simulink library "WavePlayLibBtc"  (R2022b)
settings: Solver=VariableStepAuto  StartTime=0.0  StopTime=10.0  RelTol=1e-3
values from neighbouring files (symbols this model uses):
  selectclickclack = 1    [chimes_init.m]
  TotalPeriod = 25    [chimes_init.m]
undefined symbols (not defined in the file or in its folder): Row
libraries: TuneVar x8, TOP x4, FeaturePath x1, HandyTextFile x1, RTC x1
settings Model: Creator=kl13806  LastModifiedBy=kl13806
settings SolverCC: AlgebraicLoopSolver=TrustRegion
settings DebuggingCC: UnconnectedInputMsg=warning  UnconnectedOutputMsg=warning  UnconnectedLineMsg=warning  SFMachineParentedDataDiag=warning
settings ModelReferenceCC: EnableRefExpFcnMdlSchedulingChecks=on
settings RTWCC: DLArmComputeVersion=19.05

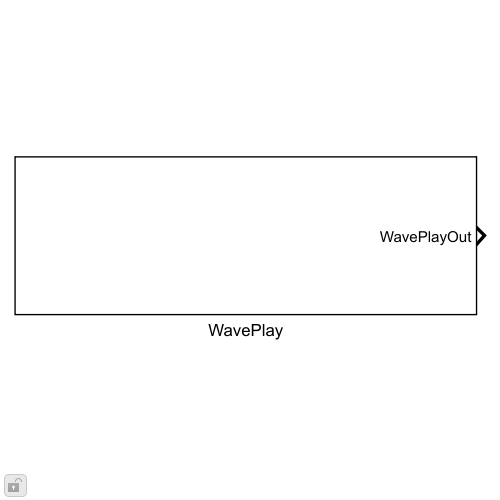
[thumbnail: Simulink's stored preview of the top-level diagram]
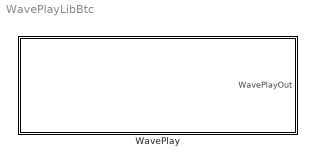
== system WavePlayLibBtc ==
  WavePlay : Subsystem  mask(Chimes WavePlay){Config=[], FeatureName=Waveplay}
      mask prompts: Config "WavePlayConfig"; FeatureName "Feature path name:"
      mask help:
      | % DESCRIPTION:
      |  Waveplay is a single-channel wave player that plays out stored waveforms.
      |   p.playControl        -  Volume and switch to start wave play
      |   p.controlState       -   Old state of playControl
      |   p.frameSize           -   Frame size
      |   p.tableLength       -   Length of the wave table
      |   p.table                   -    Wave table
      |   p.tableIndex         -    Index into wave table
      |   minVol                  -    Trigger threshold for waveplay
      mask init:
      | blkh=gcbh;
      | Config=BTConfig.Assert(blkh,Config);
      | Config.Validate();
      | BTConfig.InitSetFeatureIfPresent(blkh,'FeatureName');
      mask Callback Config: BTConfig.CallbackHideIfPresent(gcbh,{'FeatureName'});
      mask TypeOptions FeatureName: FeaturePath/FeatureName

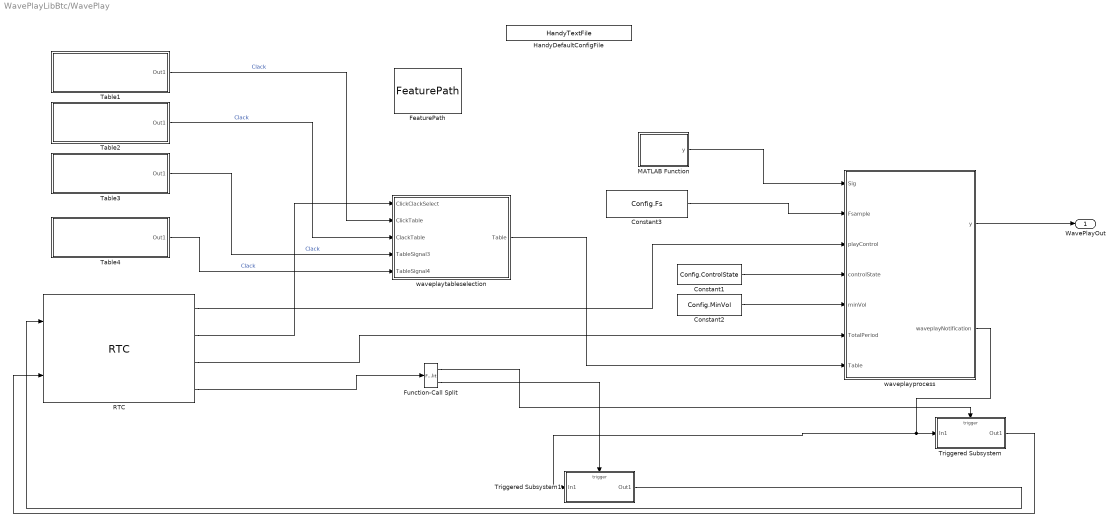
== system WavePlayLibBtc/WavePlay ==
  Constant1 : Constant  Value=Config.ControlState  OutDataTypeStr=single
  Constant2 : Constant  Value=Config.MinVol  OutDataTypeStr=single
  Constant3 : Constant  Value=Config.Fs
  FeaturePath : FeaturePath/FeaturePath  FeatureName=Waveplay  IsGroup=off  GroupNumber=-1  IsModule=off  TriggerInit=[885 274 985 341]
      settings: SourceProductName=Bose Talaria
  Function-Call Split : FunctionCallSplit  IconShape=distinctive  NumOutputPorts=2  OutputPortLayout=default
  HandyDefaultConfigFile : HandyTextFile/HandyTextFile  TemplateSource=Config  FileSuffix=Init  OpenDialogOnLoad=off  UseThisBlockName=off  AddGrandParentNamePrefix=off  TheDefaultText=|  ShowInLibBrowser=on
      | % $(FILENAME) Setup model parameters for each "Init" callback (e.g. update diagram)
      | sample_rate_in_hertz = 44100;
      | frame_size = 32;
      | sysin_channel_count = 2;
      settings: SourceProductName=Bose Talaria
  MATLAB Function : MATLAB Function  TreatAsAtomicUnit=on  mask{frameSize=Config.FrameSize}
  RTC : RTC/RTC  REQ_Priority=RTC_Mask.NormalPriority  RequestAtInit=off  EnableRequest=off  REQElemName1=WavePlayControl  REQElemType1=single  REQElemWidth1=length(Config.InitialPlayControl)  REQElemInitial1=Config.InitialPlayControl  REQElemName2=ClickClackSelect  REQElemType2=uint32  REQElemWidth2=length(selectclickclack)  REQElemInitial2=Config.InitialClickClackSelect  REQElemName3=TotalPeriod  REQElemType3=single  REQElemWidth3=length(TotalPeriod)  REQElemInitial3=Config.InitialTotalPeriodMsec  REQElemType4=uint32  REQElemWidth4=1  REQElemInitial4=[]  REQElemType5=uint32  REQElemWidth5=1  REQElemInitial5=[]  REQElemType6=uint32  REQElemWidth6=1  REQElemInitial6=[]  REQElemType7=uint32  REQElemWidth7=1  REQElemInitial7=[]  REQElemType8=uint32  REQElemWidth8=1  REQElemInitial8=[]  REQElemType9=uint32  REQElemWidth9=1  REQElemInitial9=[]  REQElemType10=uint32  REQElemWidth10=1  REQElemInitial10=[]  EnableResponse=on  EnableRSP_StatusIn=off  RSPElemType1=uint32  RSPElemWidth1=1  RSPElemType2=uint32  RSPElemWidth2=1  RSPElemType3=uint32  RSPElemWidth3=1  RSPElemType4=uint32  RSPElemWidth4=1  RSPElemType5=uint32  RSPElemWidth5=1  RSPElemType6=uint32  RSPElemWidth6=1  RSPElemType7=uint32  RSPElemWidth7=1  RSPElemType8=uint32  RSPElemWidth8=1  RSPElemType9=uint32  RSPElemWidth9=1  RSPElemType10=uint32  RSPElemWidth10=1  EnableNotification=on  EnableNTF_PrepTrig=off  NTFElemName1=WaveplayDone  NTFElemType1=uint32  NTFElemWidth1=1  NTFElemType2=uint32  NTFElemWidth2=1  NTFElemType3=uint32  NTFElemWidth3=1  NTFElemType4=uint32  NTFElemWidth4=1  NTFElemType5=uint32  NTFElemWidth5=1  NTFElemType6=uint32  NTFElemWidth6=1  NTFElemType7=uint32  NTFElemWidth7=1  NTFElemType8=uint32  NTFElemWidth8=1  NTFElemType9=uint32  NTFElemWidth9=1  NTFElemType10=uint32  NTFElemWidth10=1  MaskMessageName=RTC
      settings: SourceProductName=Bose Talaria
  Table1 : Subsystem
  Table2 : Subsystem
  Table3 : Subsystem
  Table4 : Subsystem
  Triggered Subsystem : Subsystem  TreatAsAtomicUnit=on
  Triggered Subsystem1 : Subsystem  TreatAsAtomicUnit=on
  waveplayprocess : MATLAB Function  TreatAsAtomicUnit=on
  waveplaytableselection : MATLAB Function  TreatAsAtomicUnit=on
  WavePlayOut : Outport  VectorParamsAs1DForOutWhenUnconnected=off
  wires:
  waveplayprocess/1(y) -> WavePlayOut/1
  Constant1/1 -> waveplayprocess/4(controlState)
  RTC/1 -> waveplayprocess/3(playControl)
  Constant2/1 -> waveplayprocess/5(minVol)
  Triggered Subsystem/1(Out1) -> RTC/2
  waveplayprocess/2(waveplayNotification) -> Triggered Subsystem1/1(In1), Triggered Subsystem/1(In1)
  Triggered Subsystem1/1(Out1) -> RTC/1
  RTC/4 -> Function-Call Split/1
  Function-Call Split/1 -> Triggered Subsystem/Trigger
  Function-Call Split/2 -> Triggered Subsystem1/Trigger
  Constant3/1 -> waveplayprocess/2(Fsample)
  RTC/2 -> waveplaytableselection/1(ClickClackSelect)
  Table1/1(Out1) -> waveplaytableselection/2(ClickTable)  "Clack"
  Table2/1(Out1) -> waveplaytableselection/3(ClackTable)  "Clack"
  Table3/1(Out1) -> waveplaytableselection/4(TableSignal3)  "Clack"
  Table4/1(Out1) -> waveplaytableselection/5(TableSignal4)  "Clack"
  waveplaytableselection/1(Table) -> waveplayprocess/7(Table)
  RTC/3 -> waveplayprocess/6(TotalPeriod)
  MATLAB Function/1(y) -> waveplayprocess/1(Sig)

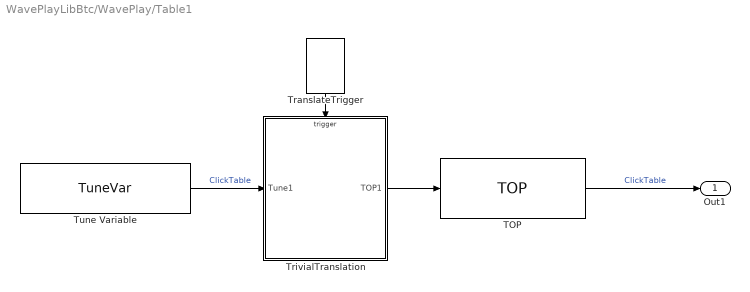
== system WavePlayLibBtc/WavePlay/Table1 ==
  TOP : TOP/TOP  TriggerInit=[440 20 585 80]  TopName=ClickTable  DataType=single  BankNumber=0  PreOverlay=false  PostOverlay=false  Role=Automatic
      settings: SourceProductName=Bose Talaria
  TranslateTrigger : TuneVar/TranslateTrigger  TriggerInit=[306 -100 344 -45]
      settings: SourceProductName=Bose Talaria
  TrivialTranslation : MATLAB Function  TreatAsAtomicUnit=on  mask(Talaria Translation){}
      mask help: This MATLAB Function Block can be automatically inserted by several automation routines. Once placed, the block is ready to accept translation logic from the model designer.
  Tune Variable : TuneVar/TuneVar  TuneName=ClickTable  SpecifyMaxSize=on  VariableDim=1 (Row)  MaxSize=[Config.MaxTableSamples 1]  TunabilityNumber=1  MinValue=[]  MaxValue=[]  TriggerInit=[20 25 190 75]  MaskValue=Config.DefaultTable1
      settings: SourceProductName=Bose Talaria
  Out1 : Outport  VectorParamsAs1DForOutWhenUnconnected=off
  wires:
  TOP/1 -> Out1/1  "ClickTable"
  Tune Variable/1 -> TrivialTranslation/1(Tune1)  "ClickTable"
  TrivialTranslation/1(TOP1) -> TOP/1
  TranslateTrigger/1 -> TrivialTranslation/Trigger

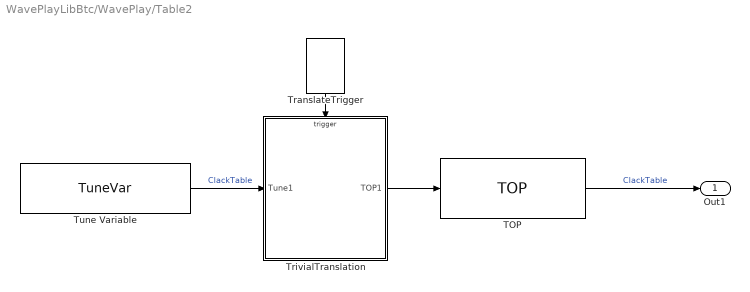
== system WavePlayLibBtc/WavePlay/Table2 ==
  TOP : TOP/TOP  TriggerInit=[440 20 585 80]  TopName=ClackTable  DataType=single  BankNumber=0  PreOverlay=false  PostOverlay=false  Role=Automatic
      settings: SourceProductName=Bose Talaria
  TranslateTrigger : TuneVar/TranslateTrigger  TriggerInit=[306 -100 344 -45]
      settings: SourceProductName=Bose Talaria
  TrivialTranslation : MATLAB Function  TreatAsAtomicUnit=on  mask(Talaria Translation){}
      mask help: This MATLAB Function Block can be automatically inserted by several automation routines. Once placed, the block is ready to accept translation logic from the model designer.
  Tune Variable : TuneVar/TuneVar  TuneName=ClackTable  SpecifyMaxSize=on  VariableDim=1 (Row)  MaxSize=[Config.MaxTableSamples 1]  TunabilityNumber=1  MinValue=[]  MaxValue=[]  TriggerInit=[20 25 190 75]  MaskValue=Config.DefaultTable2
      settings: SourceProductName=Bose Talaria
  Out1 : Outport  VectorParamsAs1DForOutWhenUnconnected=off
  wires:
  TOP/1 -> Out1/1  "ClackTable"
  Tune Variable/1 -> TrivialTranslation/1(Tune1)  "ClackTable"
  TrivialTranslation/1(TOP1) -> TOP/1
  TranslateTrigger/1 -> TrivialTranslation/Trigger

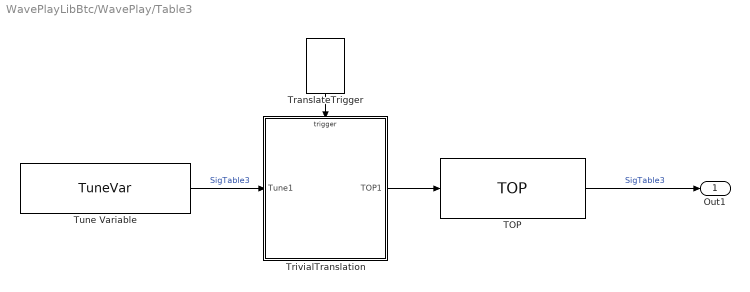
== system WavePlayLibBtc/WavePlay/Table3 ==
  TOP : TOP/TOP  TriggerInit=[440 20 585 80]  TopName=SigTable3  DataType=single  BankNumber=0  PreOverlay=false  PostOverlay=false  Role=Automatic
      settings: SourceProductName=Bose Talaria
  TranslateTrigger : TuneVar/TranslateTrigger  TriggerInit=[306 -100 344 -45]
      settings: SourceProductName=Bose Talaria
  TrivialTranslation : MATLAB Function  TreatAsAtomicUnit=on  mask(Talaria Translation){}
      mask help: This MATLAB Function Block can be automatically inserted by several automation routines. Once placed, the block is ready to accept translation logic from the model designer.
  Tune Variable : TuneVar/TuneVar  TuneName=SigTable3  SpecifyMaxSize=on  VariableDim=1 (Row)  MaxSize=[Config.MaxTableSamples 1]  TunabilityNumber=1  MinValue=[]  MaxValue=[]  TriggerInit=[20 25 190 75]  MaskValue=Config.DefaultTable3
      settings: SourceProductName=Bose Talaria
  Out1 : Outport  VectorParamsAs1DForOutWhenUnconnected=off
  wires:
  TOP/1 -> Out1/1  "SigTable3"
  Tune Variable/1 -> TrivialTranslation/1(Tune1)  "SigTable3"
  TrivialTranslation/1(TOP1) -> TOP/1
  TranslateTrigger/1 -> TrivialTranslation/Trigger

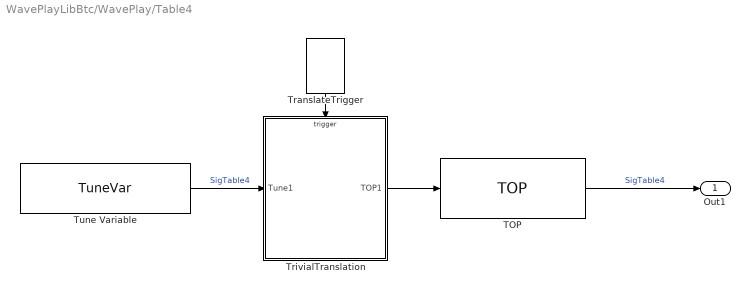
== system WavePlayLibBtc/WavePlay/Table4 ==
  TOP : TOP/TOP  TriggerInit=[440 20 585 80]  TopName=SigTable4  DataType=single  BankNumber=0  PreOverlay=false  PostOverlay=false  Role=Automatic
      settings: SourceProductName=Bose Talaria
  TranslateTrigger : TuneVar/TranslateTrigger  TriggerInit=[306 -100 344 -45]
      settings: SourceProductName=Bose Talaria
  TrivialTranslation : MATLAB Function  TreatAsAtomicUnit=on  mask(Talaria Translation){}
      mask help: This MATLAB Function Block can be automatically inserted by several automation routines. Once placed, the block is ready to accept translation logic from the model designer.
  Tune Variable : TuneVar/TuneVar  TuneName=SigTable4  SpecifyMaxSize=on  VariableDim=1 (Row)  MaxSize=[Config.MaxTableSamples 1]  TunabilityNumber=1  MinValue=[]  MaxValue=[]  TriggerInit=[20 25 190 75]  MaskValue=Config.DefaultTable4
      settings: SourceProductName=Bose Talaria
  Out1 : Outport  VectorParamsAs1DForOutWhenUnconnected=off
  wires:
  TOP/1 -> Out1/1  "SigTable4"
  Tune Variable/1 -> TrivialTranslation/1(Tune1)  "SigTable4"
  TrivialTranslation/1(TOP1) -> TOP/1
  TranslateTrigger/1 -> TrivialTranslation/Trigger

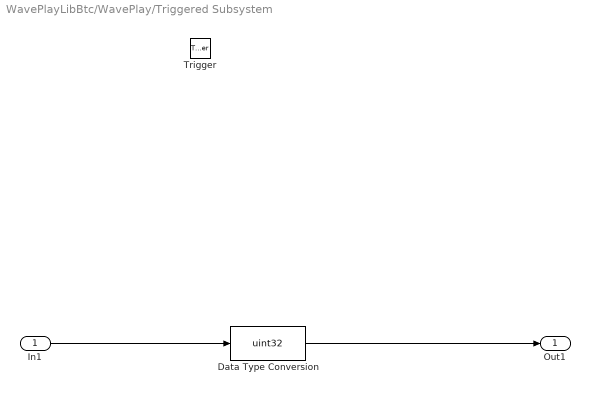
== system WavePlayLibBtc/WavePlay/Triggered Subsystem ==
  In1 : Inport
  Trigger : TriggerPort  TriggerType=function-call  VariantControl=Variant
  Data Type Conversion : DataTypeConversion  OutDataTypeStr=uint32  SaturateOnIntegerOverflow=off  RndMeth=Floor
  Out1 : Outport
  wires:
  In1/1 -> Data Type Conversion/1
  Data Type Conversion/1 -> Out1/1

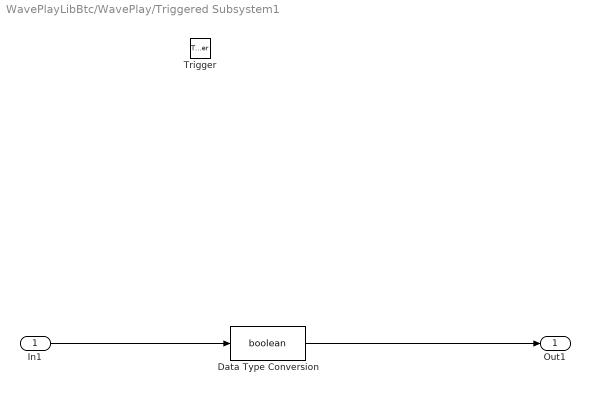
== system WavePlayLibBtc/WavePlay/Triggered Subsystem1 ==
  In1 : Inport
  Trigger : TriggerPort  TriggerType=function-call  VariantControl=Variant
  Data Type Conversion : DataTypeConversion  OutDataTypeStr=boolean  SaturateOnIntegerOverflow=off  RndMeth=Floor
  Out1 : Outport
  wires:
  Data Type Conversion/1 -> Out1/1
  In1/1 -> Data Type Conversion/1

== matlab function WavePlayLibBtc/WavePlay/waveplaytableselection ==
  data: ClickClackSelect input; Table output; ClickTable input; ClackTable input; TableSignal3 input; TableSignal4 input
function Table  = fcn(ClickClackSelect,ClickTable,ClackTable,TableSignal3,TableSignal4)
    
   MaxTableLen=single(1120.0);    
   Table = single(zeros(MaxTableLen,1));
%% Note : Maximum Table length number has been chosen based on use case of click and clack
%         signals, typically click signal is of 1079 values, and clack signal is of
%         1095 values, we round off to the nearest number in multiple of frame size.
    switch(ClickClackSelect)
        case 1 %% Click signal table selection
            Table = ClickTable;
        case 2 %% Clack signal table selection
            Table = ClackTable;
        case 3 %% Table3 signal table selection
            Table = TableSignal3;
        case 4 %% Table4 signal table selection
            Table = TableSignal4;          
    end

== matlab function WavePlayLibBtc/WavePlay/waveplayprocess ==
  data: Sig input; Fsample input; y output size=[32 1]; playControl input; controlState input; minVol input; TotalPeriod input; waveplayNotification output; Table input
function [y,waveplayNotification] = fcn(Sig,Fsample,playControl,controlState,minVol,TotalPeriod,Table)

    FrmSize= single(size(Sig,1));
    Fsamp= Fsample(1,1);
    
    waveplayNotification =single(0.0);
    persistent OutStore ;
    persistent waveplayDone;
    persistent ctlState;
    persistent tableIndex;
    persistent SilencePeriodCounter;
    Numchannels = size(Table,2);
    tableLength = size(Table,1);
    TablePeriod = (tableLength/Fsamp)*1000;
    quantum_ms  = 1000 * FrmSize / Fsamp;
    SilencePeriod= TotalPeriod - TablePeriod;
    
    if(isempty(OutStore))
        SilencePeriodCounter = ceil(SilencePeriod/quantum_ms);
    end

    if(isempty(OutStore))
         OutStore = single(zeros(FrmSize,Numchannels));        
    end
    if(isempty(ctlState))
        ctlState = controlState;% single(0.0);
    end
    if(isempty(tableIndex))
        tableIndex = single(0.0);
    end
    if(isempty(waveplayDone))
        waveplayDone =single(0.0);
    end
    
    if (playControl < minVol)    % playControl == 0
        OutStore(:,1:Numchannels) = zeros(FrmSize, 1);   
    else                           % playControl ~= 0
    % start wave play at the rising edge of playControl signal
    % assuming p has been properly initialized before rising edge occurs
        if((playControl - ctlState) > minVol)      % trigger detected
            % playControl also acts as playing volume     
            OutStore(:,1:Numchannels) = playControl .* Table(1:FrmSize);
            tableIndex = FrmSize;  % update tabelIndex after outputing the 1st frame
        else       %  playControl = controlState (both >= minVol)
            i = tableIndex;
            %if(i >= tableLength)
            if((tableLength-tableIndex)<FrmSize)
                %We do reset here, compared to BDSP implementation
                tableIndex = single(0.0);
                waveplayDone=single(1.0);
                i=single(0.0);
            end
            if (i < tableLength)   % continuation frame
                OutStore(:,1:Numchannels) = playControl .* Table(i+1:i+FrmSize);
                tableIndex = i + FrmSize;   % don't wrap around, o/w, next condition won't be met
            else        % i >= p.tableLength, wave table done
                OutStore(:,1:Numchannels) = zeros(FrmSize, 1);   
                % don't update tableIndex to keep the condition "i >= tableLength" valid
                % TableIndex will be reset when next trigger arrives
            end  
        end
   end
    ctlState = playControl;   % save previous state
    if(waveplayDone)
        %This is a wrap around case when table is finished,if we have
        %silent period>0 then only we send zeros to microcontroller
        %otherwise we need to wrap around to table values after we complete
        %reading table 
        if(SilencePeriodCounter>0)% To avoid boundary condition
            SilencePeriodCounter=SilencePeriodCounter-1;
            OutStore(:,1:Numchannels) = zeros(FrmSize, 1);
            tableIndex = single(0.0);
        end
      if(~SilencePeriodCounter)
        waveplayDone=single(0.0);  
        %Now that we are done with check of click/clack table finished,
        %And also the silence period is completed,notify to micro.
        waveplayNotification =single(1.0);
        SilencePeriodCounter = ceil(SilencePeriod/quantum_ms);        
      end
    end %% waveplayDone
 y = OutStore;

== matlab function WavePlayLibBtc/WavePlay/MATLAB Function ==
  data: y output size=[frameSize 1]; frameSize parameter
function y = fcn(frameSize)
% zero padding 
y = zeros(frameSize,1);

== matlab function WavePlayLibBtc/WavePlay/Table2/TrivialTranslation ==
  data: TOP1 output; Tune1 input
  events: trigger input FUNCTION_CALL_EVENT
function TOP1  = fcn(Tune1)
%#codegen

% ----- To access TuneVar maximum size, current size, and current value:
%   Note: TuneVar signals arrive with exposed variable size information.
%         The expressions below illustrate for the "Tune1" input argument.
%
%   size(Tune1.Value) : the maximum possible size of the Tune1 variable
%
%   Tune.Size   : the current size of *valid* data in Tune1.Value
%
%   Tune1.Size(1) : Number of rows present in Tune1 - this does not vary.
%
%   Tune1.Size(2) : Number of columns currently valid in Tune1 - this is
%       the variable part of size that can change (if allowed by TuneVar).
%
%   Tune1.Value : the current value of the tune variable... but end-padded 
%       to the maximum available size with undefined/invalid data.
%
%   numel(Tune1.Value) : another way of looking at the maximum number of
%       elements that could arrive in Tune1.Value
%
% ----- To register an error, use the following method (works like printf):
%   TranslateError( <format string>, <arguments ... )
%   ... this error will cause the build process to abort.
% ----- For warnings (works like printf):
%   TranslateWarning( <format string>, <arguments ... )
%   ... this warning will not set the translation engine error state.

% A trivial pass-through translation looks like this:
TOP1 = Tune1.Value;

== matlab function WavePlayLibBtc/WavePlay/Table3/TrivialTranslation ==
  data: TOP1 output; Tune1 input
  events: trigger input FUNCTION_CALL_EVENT
function TOP1  = fcn(Tune1)
%#codegen

% ----- To access TuneVar maximum size, current size, and current value:
%   Note: TuneVar signals arrive with exposed variable size information.
%         The expressions below illustrate for the "Tune1" input argument.
%
%   size(Tune1.Value) : the maximum possible size of the Tune1 variable
%
%   Tune.Size   : the current size of *valid* data in Tune1.Value
%
%   Tune1.Size(1) : Number of rows present in Tune1 - this does not vary.
%
%   Tune1.Size(2) : Number of columns currently valid in Tune1 - this is
%       the variable part of size that can change (if allowed by TuneVar).
%
%   Tune1.Value : the current value of the tune variable... but end-padded 
%       to the maximum available size with undefined/invalid data.
%
%   numel(Tune1.Value) : another way of looking at the maximum number of
%       elements that could arrive in Tune1.Value
%
% ----- To register an error, use the following method (works like printf):
%   TranslateError( <format string>, <arguments ... )
%   ... this error will cause the build process to abort.
% ----- For warnings (works like printf):
%   TranslateWarning( <format string>, <arguments ... )
%   ... this warning will not set the translation engine error state.

% A trivial pass-through translation looks like this:
TOP1 = Tune1.Value;

== matlab function WavePlayLibBtc/WavePlay/Table4/TrivialTranslation ==
  data: TOP1 output; Tune1 input
  events: trigger input FUNCTION_CALL_EVENT
function TOP1  = fcn(Tune1)
%#codegen

% ----- To access TuneVar maximum size, current size, and current value:
%   Note: TuneVar signals arrive with exposed variable size information.
%         The expressions below illustrate for the "Tune1" input argument.
%
%   size(Tune1.Value) : the maximum possible size of the Tune1 variable
%
%   Tune.Size   : the current size of *valid* data in Tune1.Value
%
%   Tune1.Size(1) : Number of rows present in Tune1 - this does not vary.
%
%   Tune1.Size(2) : Number of columns currently valid in Tune1 - this is
%       the variable part of size that can change (if allowed by TuneVar).
%
%   Tune1.Value : the current value of the tune variable... but end-padded 
%       to the maximum available size with undefined/invalid data.
%
%   numel(Tune1.Value) : another way of looking at the maximum number of
%       elements that could arrive in Tune1.Value
%
% ----- To register an error, use the following method (works like printf):
%   TranslateError( <format string>, <arguments ... )
%   ... this error will cause the build process to abort.
% ----- For warnings (works like printf):
%   TranslateWarning( <format string>, <arguments ... )
%   ... this warning will not set the translation engine error state.

% A trivial pass-through translation looks like this:
TOP1 = Tune1.Value;

== matlab function WavePlayLibBtc/WavePlay/Table1/TrivialTranslation ==
  data: TOP1 output; Tune1 input
  events: trigger input FUNCTION_CALL_EVENT
function TOP1  = fcn(Tune1)
%#codegen

% ----- To access TuneVar maximum size, current size, and current value:
%   Note: TuneVar signals arrive with exposed variable size information.
%         The expressions below illustrate for the "Tune1" input argument.
%
%   size(Tune1.Value) : the maximum possible size of the Tune1 variable
%
%   Tune.Size   : the current size of *valid* data in Tune1.Value
%
%   Tune1.Size(1) : Number of rows present in Tune1 - this does not vary.
%
%   Tune1.Size(2) : Number of columns currently valid in Tune1 - this is
%       the variable part of size that can change (if allowed by TuneVar).
%
%   Tune1.Value : the current value of the tune variable... but end-padded 
%       to the maximum available size with undefined/invalid data.
%
%   numel(Tune1.Value) : another way of looking at the maximum number of
%       elements that could arrive in Tune1.Value
%
% ----- To register an error, use the following method (works like printf):
%   TranslateError( <format string>, <arguments ... )
%   ... this error will cause the build process to abort.
% ----- For warnings (works like printf):
%   TranslateWarning( <format string>, <arguments ... )
%   ... this warning will not set the translation engine error state.

% A trivial pass-through translation looks like this:
TOP1 = Tune1.Value;
